simulink model "ggPertValidation"  (R2024b)
settings: Solver=VariableStepAuto  StartTime=0.0  StopTime=10.0  RelTol=1e-3
values from neighbouring files (symbols this model uses):
  J = diag([0.4 0.6 0.8])    [validationGGpert.m]
  mu = constant.mu    [validateMagField.m]    (also in validationGGpert.m)
  n_B = n_B/norm(n_B)    [validationGGpert.m]
  rNorm = Re + 600    [validateMagField.m]    (also in validationGGpert.m)
libraries: matrix_library x1
settings Model: Creator=ricca  LastModifiedBy=ricca

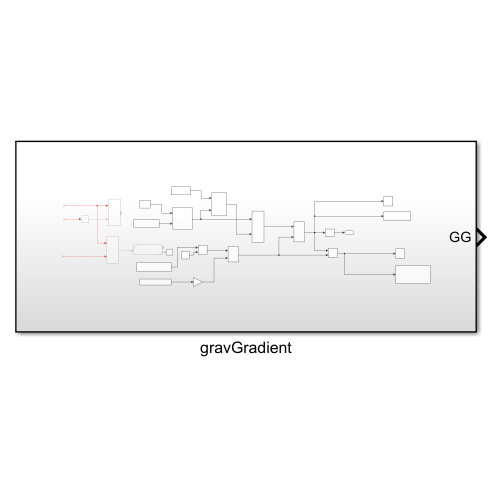
[thumbnail: Simulink's stored preview of the top-level diagram]
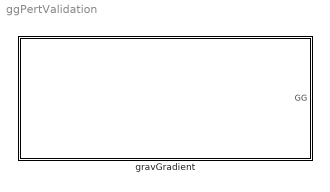
== system ggPertValidation ==
  gravGradient : Subsystem

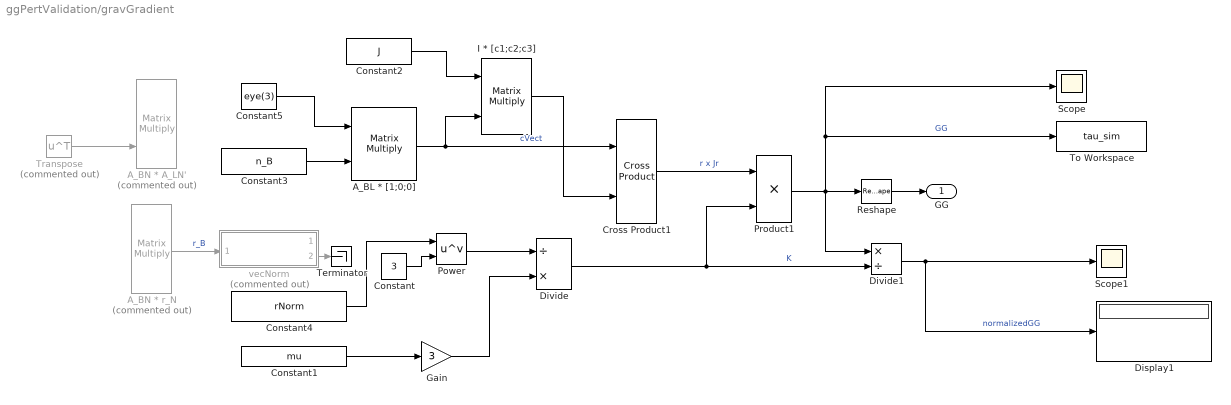
== system ggPertValidation/gravGradient ==
  A_BL * [1;0;0] : Product  Multiplication=Matrix(*)
  A_BN * A_LN' : Product  Commented=on  Multiplication=Matrix(*)
  A_BN * r_N : Product  Commented=on  Multiplication=Matrix(*)
  Constant : Constant  Value=3
  Constant1 : Constant  Value=mu
  Constant2 : Constant  Value=J
  Constant3 : Constant  Value=n_B
  Constant4 : Constant  Value=rNorm
  Constant5 : Constant  Value=eye(3)
  Cross Product1 : matrix_library/Cross Product
  Display1 : Display
  Divide : Product  Inputs=/*
  Divide1 : Product  Inputs=*/
  Gain : Gain  Gain=3
  I * [c1;c2;c3] : Product  Multiplication=Matrix(*)
  Power : Math  Operator=pow
  Product1 : Product
  Reshape : Reshape
  Scope : Scope
  Scope1 : Scope
  Terminator : Terminator
  To Workspace : ToWorkspace  VariableName=tau_sim  SampleTime=-1
  Transpose : Math  Commented=on  Operator=transpose
  vecNorm : Subsystem  Commented=on  ReferencedSubsystem=vecNorm
  GG : Outport
  wires:
  Constant3/1 -> A_BL * [1;0;0]/2
  A_BL * [1;0;0]/1 -> Cross Product1/1, I * [c1;c2;c3]/2  "cVect"
  Product1/1 -> To Workspace/1, Scope/1, Divide1/1, Reshape/1  "GG"
  Transpose/1 -> A_BN * A_LN'/2
  ? -> A_BN * A_LN'/1, A_BN * r_N/1  "ABN"
  ? -> Transpose/1  "ALN"
  Divide/1 -> Divide1/2, Product1/2  "K"
  Power/1 -> Divide/1
  Constant/1 -> Power/2
  ? -> A_BN * r_N/2  "rN"
  A_BN * r_N/1 -> vecNorm/1  "r_B"
  Constant1/1 -> Gain/1
  Gain/1 -> Divide/2
  vecNorm/2 -> Terminator/1
  I * [c1;c2;c3]/1 -> Cross Product1/2
  Constant2/1 -> I * [c1;c2;c3]/1
  Cross Product1/1 -> Product1/1  "r x Jr"
  Reshape/1 -> GG/1
  Constant4/1 -> Power/1
  Divide1/1 -> Display1/1, Scope1/1  "normalizedGG"
  Constant5/1 -> A_BL * [1;0;0]/1
